simulink model "Grid_FormingVSG_PMSG"  (R2024b)
settings: Solver=ode3  StartTime=0.0  StopTime=44.2  FixedStep=1e-6  RelTol=1e-3  EnableMultiTasking=on
InitFcn:
  | mdlFile = get_param(bdroot,'FileName');
  | mdlDir = fileparts(mdlFile);
  | dtime=4e-6;
  | Ts_step=1e-6;
  | run(fullfile(mdlDir,'GFM_MWT_Nonlinear_Params.m'));
values from neighbouring files (symbols this model uses):
  D_aero = T_aero0 / omega_m0    (= 101321.183642)    [GFM_MWT_Nonlinear_Params.m]    (also in GFM_MWT_Nonlinear_Params_5MW_Liu2024.m = T_aero0/omega_m0)
  D_g = 0.005 * D_aero    (= 506.605918212)    [GFM_MWT_Nonlinear_Params.m]    (also in GFM_MWT_Nonlinear_Params_5MW_Liu2024.m = p5.D_g)
  D_sh = evalin('base','D_sh_override')    [GFM_MWT_Nonlinear_Params.m]    (also in GFM_MWT_Nonlinear_Params_5MW_Liu2024.m = shaft_damping_scale*D_sh)
  D_t = 0.005 * D_aero    (= 506.605918212)    [GFM_MWT_Nonlinear_Params.m]    (also in GFM_MWT_Nonlinear_Params_5MW_Liu2024.m = p5.D_t)
  J_g = 1.83750e5    (= 183750)    [GFM_MWT_Nonlinear_Params.m]    (also in GFM_MWT_Nonlinear_Params_5MW_Liu2024.m = p5.J_g)
  J_t = 8.0 * J_g    (= 1470000)    [GFM_MWT_Nonlinear_Params.m]    (also in GFM_MWT_Nonlinear_Params_5MW_Liu2024.m = p5.J_t)
  K_sh = J_eq * w_sh_init_guess^2    (= 6448141.54205)    [GFM_MWT_Nonlinear_Params.m]    (also in GFM_MWT_Nonlinear_Params_5MW_Liu2024.m = p5.K_sh)
  K_v_aero = 3 * T_aero0 / v_w0    (= 79577.4715459)    [GFM_MWT_Nonlinear_Params.m]    (also in GFM_MWT_Nonlinear_Params_5MW_Liu2024.m = 3*T_aero0/v_w0)
  omega_m0 = 2*pi*30/60    (= 3.14159265359)    [GFM_MWT_Nonlinear_Params.m]    (also in GFM_MWT_Nonlinear_Params_5MW_Liu2024.m = p5.omega_m0)
  T_aero0 = T_e0    (= 318309.886184)    [GFM_MWT_Nonlinear_Params.m]    (also in GFM_MWT_Nonlinear_Params_5MW_Liu2024.m = T_e0)
  theta_tw0 = T_e0 / K_sh    (= 0.0493645935202)    [GFM_MWT_Nonlinear_Params.m]    (also in GFM_MWT_Nonlinear_Params_5MW_Liu2024.m = T_e0/K_sh)
  v_w0 = 12.0    (= 12)    [GFM_MWT_Nonlinear_Params.m]    (also in GFM_MWT_Nonlinear_Params_5MW_Liu2024.m = p5.v_w0)
  wind_step_mps = evalin('base','wind_step_mps_override')    [GFM_MWT_Nonlinear_Params.m]    (also in GFM_MWT_Nonlinear_Params_5MW_Liu2024.m)
  wind_step_time = 1.50    (= 1.5)    [GFM_MWT_Nonlinear_Params.m]    (also in GFM_MWT_Nonlinear_Params_5MW_Liu2024.m = evalin('base','wind_step_time_override'))
undefined symbols (not defined in the file or in its folder): DiscIntNeverNeededParam
libraries: spsSeriesRLCBranchLib x10, spsVoltageMeasurementLib x7, spsCurrentMeasurementLib x6, spsACVoltageSourceLib x3, spsUniversalBridgeLib x2, powerlib_extras x2, spsControlledCurrentSourceLib x2, spsGroundLib x1, simulink x1, spsThreePhaseBreakerLib x1, spspowerguiLib x1
settings Model: Creator=Administrator  LastModifiedBy=Lenovo
settings SolverCC: AlgebraicLoopSolver=TrustRegion
settings DataIOCC: LimitDataPoints=on  LoadInitialState=on  SaveFinalState=on  SaveFormat=Array  SignalLoggingSaveFormat=ModelDataLogs
settings OptimizationCC: ExpressionDepthLimit=2147483647  LifeSpan=inf
settings DebuggingCC: UnderspecifiedInitializationDetection=Classic  MergeDetectMultiDrivingBlocksExec=none  SolverPrmCheckMsg=warning  FcnCallInpInsideContextMsg=warning  UnconnectedInputMsg=warning  UnconnectedOutputMsg=warning  UnconnectedLineMsg=warning  StateNameClashWarn=warning  SFUnexpectedBacktrackingDiag=warning  SFNoUnconditionalDefaultTransitionDiag=warning  SFExecutionAtInitializationDiag=none  ArithmeticOperatorsInVariantConditions=warning
settings HardwareCC: ProdBitPerPointer=32  ProdBitPerSizeT=32  ProdBitPerPtrDiffT=32  ProdLargestAtomicFloat=None  ProdIntDivRoundTo=Undefined  ProdEndianess=Unspecified  ProdWordSize=32  ProdHWDeviceType=32-bit Generic
settings ModelReferenceCC: EnableRefExpFcnMdlSchedulingChecks=on  PropagateSignalLabelsOutOfModel=off
settings SFSimCC: SimUseLocalCustomCode=off  CustomCodeUndefinedFunction=UseInterfaceOnly
settings RTWCC: RTWUseLocalCustomCode=off  GPUComputeCapability=3.5
settings CodeAppCC: StateflowObjectComments=on
settings GRTTargetCC: TargetLangStandard=C89/C90 (ANSI)
settings ConfigComp: CovMetricSettings=dw  CovSaveCumulativeToWorkspaceVar=on  CovSaveSingleToWorkspaceVar=on  CovExternalEMLEnable=off
settings SimscapeCC: SimscapeNormalizeSystem=off

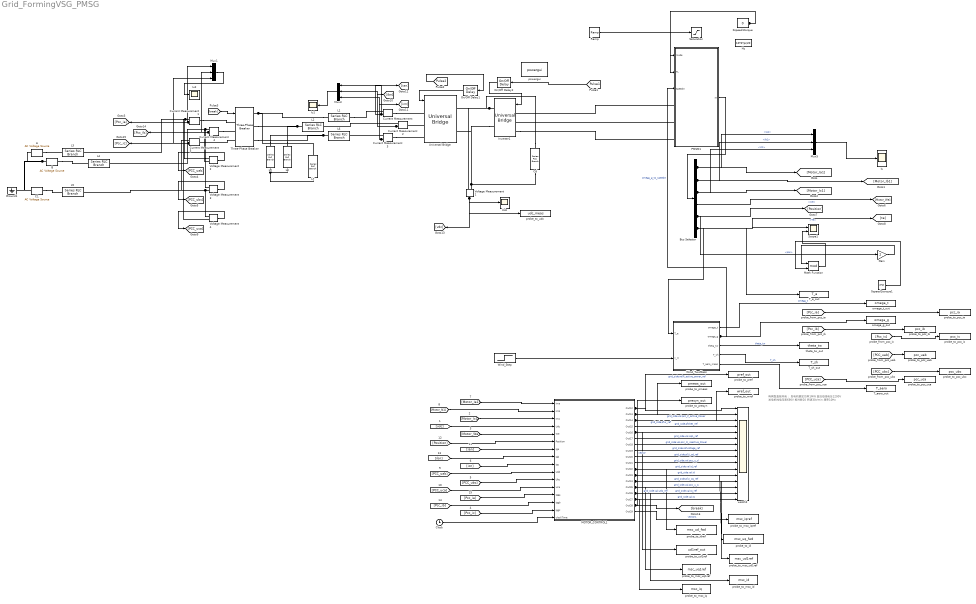
== system Grid_FormingVSG_PMSG ==
  note: 构网型直驱风电：
      | 发电机额定功率1MW
      | 直流母线电压1200V
      | 发电机线电压是690V
      | 极对数20
      | 转速30r/min
      | 频率10Hz
  0speed1torque : Constant  Value=0
  0speed1torque1 : Constant  Value=2*pi
  A : spsACVoltageSourceLib/AC Voltage Source  Amplitude=563  Phase=10  Frequency=50  SampleTime=0  Measurements=None  BusType=swing  Pref=10e3  Qref=0  Qmin=-inf  Qmax=+inf
  B : spsACVoltageSourceLib/AC Voltage Source  Amplitude=563  Phase=-110  Frequency=50  SampleTime=0  Measurements=None  BusType=swing  Pref=10e3  Qref=0  Qmin=-inf  Qmax=+inf
  Bus Selector : BusSelector  OutputSignals=Statormeasurements.ia1,Statormeasurements.ib1,Statormeasurements.ic1,Mechanical.we,Mechanical.pos,Mechanical.Te
  C1 : spsACVoltageSourceLib/AC Voltage Source  Amplitude=563  Phase=130  Frequency=50  SampleTime=0  Measurements=None  BusType=swing  Pref=10e3  Qref=0  Qmin=-inf  Qmax=+inf
  Cd : spsSeriesRLCBranchLib/Series RLC Branch  LConnTagsString=__new0  RConnTagsString=__new0  BranchType=C  Resistance=100  Inductance=1e-3  SetiL0=off  InitialCurrent=0  Capacitance=0.03  Setx0=on  InitialVoltage=1200  Measurements=None
  Clock : Clock
  Current Measurement{,1..5} (6 alike) : spsCurrentMeasurementLib/Current Measurement  PhasorSimulation=off  OutputType=Complex  PSBequivalent=0
  Gain : Gain  Gain=2
  Ground1 : spsGroundLib/Ground  LConnTagsString=a
  Hz : Constant  Value=10*2*pi/20
  Inverter1 : spsUniversalBridgeLib/Universal Bridge  Arms=3  SnubberResistance=1e5  SnubberCapacitance=inf  Device=IGBT / Diodes  Ron=1e-3  Lon=0  ForwardVoltages="[0  0]"  ForwardVoltage=0  GTOparameters=[ 10e-6 , 20e-6 ]  IGBTparameters=[ 1e-6 , 2e-6 ]  Measurements=None  Measurements_2=None  converterType=Rectifier
  Iu : Scope
  Iu1 : Scope
  Iu2 : Scope
  L1 : spsSeriesRLCBranchLib/Series RLC Branch  LConnTagsString=__new0  RConnTagsString=__new0  BranchType=RL  Resistance=0.0002  Inductance=120e-6  SetiL0=off  InitialCurrent=0  Capacitance=2e-3  Setx0=off  InitialVoltage=0  Measurements=None
  L2 : spsSeriesRLCBranchLib/Series RLC Branch  LConnTagsString=__new0  RConnTagsString=__new0  BranchType=RL  Resistance=0.0002  Inductance=120e-6  SetiL0=off  InitialCurrent=0  Capacitance=2e-3  Setx0=off  InitialVoltage=0  Measurements=None
  L3 : spsSeriesRLCBranchLib/Series RLC Branch  LConnTagsString=__new0  RConnTagsString=__new0  BranchType=L  Resistance=0.0083  Inductance=0.48e-3  SetiL0=off  InitialCurrent=0  Capacitance=2e-3  Setx0=off  InitialVoltage=0  Measurements=None
  L4 : spsSeriesRLCBranchLib/Series RLC Branch  LConnTagsString=__new0  RConnTagsString=__new0  BranchType=L  Resistance=0.0083  Inductance=0.48e-3  SetiL0=off  InitialCurrent=0  Capacitance=2e-3  Setx0=off  InitialVoltage=0  Measurements=None
  L5 : spsSeriesRLCBranchLib/Series RLC Branch  LConnTagsString=__new0  RConnTagsString=__new0  BranchType=L  Resistance=0.1  Inductance=0.48e-3  SetiL0=off  InitialCurrent=0  Capacitance=2e-3  Setx0=off  InitialVoltage=0  Measurements=None
  L6 : spsSeriesRLCBranchLib/Series RLC Branch  LConnTagsString=__new0  RConnTagsString=__new0  BranchType=RL  Resistance=0.0002  Inductance=120e-6  SetiL0=off  InitialCurrent=0  Capacitance=2e-3  Setx0=off  InitialVoltage=0  Measurements=None
  L7 : spsSeriesRLCBranchLib/Series RLC Branch  LConnTagsString=__new0  RConnTagsString=__new0  BranchType=C  Resistance=0.0002  Inductance=0.00025  SetiL0=off  InitialCurrent=0  Capacitance=55e-6  Setx0=off  InitialVoltage=0  Measurements=None
  L8 : spsSeriesRLCBranchLib/Series RLC Branch  LConnTagsString=__new0  RConnTagsString=__new0  BranchType=C  Resistance=0.0002  Inductance=0.00025  SetiL0=off  InitialCurrent=0  Capacitance=55e-6  Setx0=off  InitialVoltage=0  Measurements=None
  L9 : spsSeriesRLCBranchLib/Series RLC Branch  LConnTagsString=__new0  RConnTagsString=__new0  BranchType=C  Resistance=0.0002  Inductance=0.00025  SetiL0=off  InitialCurrent=0  Capacitance=55e-6  Setx0=off  InitialVoltage=0  Measurements=None
  MOTOR_CONTROL1 : Subsystem  mask{Pref=1000000, Qref=0, ReferenceACVoltage=563, ReferenceDCVoltage=1000}
      mask prompts: Pref "Active Power"; Qref "Reactive Power"; ReferenceACVoltage "Reference AC Voltage"; ReferenceDCVoltage "Reference DC Voltage"
  Math Function : Math  Operator=mod  SignedPower=on
  Mux1 : Mux  Inputs=3
  Mux3 : Mux  Inputs=3
  Mux5 : Mux  Inputs=3
  On/Off Delay1 : powerlib_extras/Control  Blocks/On//Off Delay  type_delay=On delay  delay=dtime  ic=0
  On/Off Delay2 : powerlib_extras/Control  Blocks/On//Off Delay  type_delay=On delay  delay=dtime  ic=0
  PMSM1 : Subsystem  mask{Rpass=1e2, Cpass=1e-6, Flux=8.64, Rs=0.0122, Lq=0.00105, Ld=0.00105, pairs=20, J=183750, Bw=0.001}
  Ramp : simulink/Sources/Ramp  slope=1000  start=0.2  InitialOutput=0
  Saturation : Saturate  UpperLimit=9.55
  Scope1 : Scope  NumInputPorts=2
  T_aero_out : ToWorkspace  VariableName=T_aero  SaveFormat=Timeseries  SampleTime=-1
      settings: Decimation=mech_log_decimation
  T_e_out : ToWorkspace  VariableName=T_e  SaveFormat=Timeseries  SampleTime=-1
      settings: Decimation=mech_log_decimation
  T_sh_out : ToWorkspace  VariableName=T_sh  SaveFormat=Timeseries  SampleTime=-1
      settings: Decimation=mech_log_decimation
  Three-Phase Breaker : spsThreePhaseBreakerLib/Three-Phase Breaker  InitialState=closed  SwitchA=on  SwitchB=on  SwitchC=on  SwitchTimes=[3 3.15]  External=on  BreakerResistance=0.0001  SnubberResistance=1e6  SnubberCapacitance=inf  Measurements=None
  Udc : Scope
  Universal Bridge : spsUniversalBridgeLib/Universal Bridge  Arms=3  SnubberResistance=1e5  SnubberCapacitance=inf  Device=MOSFET / Diodes  Ron=1e-3  Lon=0  ForwardVoltages="[  0  0  ]"  ForwardVoltage=0  GTOparameters=[ 10e-6 , 20e-6 ]  IGBTparameters=[ 1e-6 , 2e-6 ]  Measurements=None  Measurements_2=None  converterType=Rectifier
  Voltage Measurement{1..4} (4 alike) : spsVoltageMeasurementLib/Voltage Measurement  PhasorSimulation=off  OutputType=Complex  PSBequivalent=0
  Wind_Step : Step  Time=wind_step_time  Before=v_w0  After=v_w0 + wind_step_mps  SampleTime=0
  Wind_TwoMass : Subsystem
  omega_g_out : ToWorkspace  VariableName=omega_g  SaveFormat=Timeseries  SampleTime=-1
      settings: Decimation=mech_log_decimation
  omega_t_out : ToWorkspace  VariableName=omega_t  SaveFormat=Timeseries  SampleTime=-1
      settings: Decimation=mech_log_decimation
  powergui : spspowerguiLib/powergui  SimulationMode=Discrete  SampleTime=Ts_step  frequency=60  Iterations=50  frequencyindice=0  Pbase=100e6  ErrMax=1e-4  UnitsV=kV  UnitsW=MW  buscounter=0  FunctionMessages=off  echomessages=off  EnableUseOfTLC=off  CurrentSourceSwitches=off  DisableSnubberDevices=off  DisableRonSwitches=off  DisableVfSwitches=off  DisplayEquations=off  AutomaticDiscreteSolvers=off  SolverType=Tustin  Interpol=off  ExternalGateDelay=off  methode=off  Ts=0  x0status=blocks  SPID=off  SwTol=0  HookPort=off  NonlinearTolerance=1e-4  nMaxIteration=100  ContinueOnMaxIteration=off  RestoreLinks=warning  ResistiveCurrentMeasurement=off  Frange=[0:2:500]  Ylog=off  Xlog=on  ShowGrid=off  save=off  variable=ZData  structure=Iu1  ZoomFFT=off  StartTime=3.5  cycles=3  DisplayStyle=4  fundamental=50  FreqAxis=off  MaxFrequency=4000  frequencyindicesteady=1  RmsSteady=1  display=off
  probe_to_id : ToWorkspace  VariableName=msc_uq_fwd  SaveFormat=Structure With Time  SampleTime=-1
  probe_to_idref : ToWorkspace  VariableName=msc_ud_fwd  SaveFormat=Structure With Time  SampleTime=-1
  probe_to_msc_id : ToWorkspace  VariableName=msc_id  SaveFormat=Timeseries
  probe_to_msc_iq : ToWorkspace  VariableName=msc_iq  SaveFormat=Timeseries
  probe_to_msc_iqref : ToWorkspace  VariableName=msc_iqref  SaveFormat=Timeseries
  probe_to_msc_ud1ref : ToWorkspace  VariableName=msc_ud1ref  SaveFormat=Timeseries
  probe_to_msc_uq1ref : ToWorkspace  VariableName=msc_uq1ref  SaveFormat=Timeseries
  probe_to_pcc_ia : ToWorkspace  VariableName=pcc_ia  SaveFormat=Timeseries  SampleTime=-1
      settings: Decimation=100
  probe_to_pcc_ib : ToWorkspace  VariableName=pcc_ib  SaveFormat=Timeseries  SampleTime=-1
      settings: Decimation=100
  probe_to_pcc_ic : ToWorkspace  VariableName=pcc_ic  SaveFormat=Timeseries  SampleTime=-1
      settings: Decimation=100
  probe_to_pcc_uab : ToWorkspace  VariableName=pcc_uab  SaveFormat=Timeseries  SampleTime=-1
      settings: Decimation=100
  probe_to_pcc_ubc : ToWorkspace  VariableName=pcc_ubc  SaveFormat=Timeseries  SampleTime=-1
      settings: Decimation=100
  probe_to_pcc_uca : ToWorkspace  VariableName=pcc_uca  SaveFormat=Timeseries  SampleTime=-1
      settings: Decimation=100
  probe_to_pmeas : ToWorkspace  VariableName=pmeas_out  SaveFormat=Timeseries  SampleTime=-1
      settings: Decimation=100
  probe_to_pref : ToWorkspace  VariableName=pref_out  SaveFormat=Timeseries  SampleTime=-1
      settings: Decimation=100
  probe_to_presyn : ToWorkspace  VariableName=presyn_out  SaveFormat=Timeseries  SampleTime=-1
      settings: Decimation=100
  probe_to_ud1ref : ToWorkspace  VariableName=ud1ref_out  SaveFormat=Structure With Time  SampleTime=-1
  probe_to_udc : ToWorkspace  VariableName=udc_meas  SaveFormat=Timeseries  SampleTime=-1
      settings: Decimation=100
  probe_to_wref : ToWorkspace  VariableName=wref_out  SaveFormat=Timeseries  SampleTime=-1
      settings: Decimation=100
  theta_tw_out : ToWorkspace  VariableName=theta_tw  SaveFormat=Timeseries  SampleTime=-1
      settings: Decimation=mech_log_decimation
  watch2 : Scope  NumInputPorts=16
  wires:
  MOTOR_CONTROL1/18(Out29) -> probe_to_msc_iqref/1  "vector1"
  Wind_TwoMass/5(T_aero_meas) -> T_aero_out/1
  [PCC_uca] -> probe_to_pcc_uca/1
  [PCC_ubc] -> probe_to_pcc_ubc/1
  [PCC_uab] -> probe_to_pcc_uab/1
  [Pcc_ic] -> probe_to_pcc_ic/1
  [Pcc_ib] -> probe_to_pcc_ib/1
  [Pcc_ia] -> probe_to_pcc_ia/1
  Wind_TwoMass/4(T_sh) -> T_sh_out/1  "T_sh"
  Wind_TwoMass/3(theta_tw) -> theta_tw_out/1  "theta_tw"
  Wind_TwoMass/1(omega_t) -> omega_t_out/1  "omega_t"
  Wind_TwoMass/2(omega_g) -> PMSM1/3(Speedin), omega_g_out/1  "omega_g_to_speedin"
  Wind_Step/1 -> Wind_TwoMass/2(v_w)
  Current Measurement3/1 -> Mux3/3, [icn]
  Current Measurement2/1 -> [ibn], Mux3/2
  Current Measurement/1 -> [ian], Mux3/1
  Current Measurement5/1 -> [Pcc_ic], Mux1/3
  Current Measurement4/1 -> [Pcc_ib], Mux1/2
  Current Measurement1/1 -> [Pcc_ia], Mux1/1
  Mux1/1 -> Iu2/1
  [break] -> Three-Phase Breaker/1
  MOTOR_CONTROL1/17(Out28) -> probe_to_presyn/1, [break]  "vector"
  Clock/1 -> MOTOR_CONTROL1/16(clockTime)
  [Pcc_ic] -> MOTOR_CONTROL1/15(Iggc)
  [Pcc_ib] -> MOTOR_CONTROL1/14(Iggb)
  [Pcc_ia] -> MOTOR_CONTROL1/13(Igga)
  Voltage Measurement3/1 -> [PCC_ubc]
  Voltage Measurement4/1 -> [PCC_uca]
  Voltage Measurement2/1 -> [PCC_uab]
  [ian] -> MOTOR_CONTROL1/7(Iga)
  [PCC_ubc] -> MOTOR_CONTROL1/11(Ubc)
  [PCC_uca] -> MOTOR_CONTROL1/12(Uca)
  [ibn] -> MOTOR_CONTROL1/8(Igb)
  [PCC_uab] -> MOTOR_CONTROL1/10(Uab)
  [icn] -> MOTOR_CONTROL1/9(Igc)
  On/Off Delay1/1 -> Universal Bridge/1
  [Pulse2] -> On/Off Delay1/1
  Mux3/1 -> Iu1/1
  Voltage Measurement1/1 -> Udc/1, [vdc], probe_to_udc/1
  [Motor_Ia1] -> MOTOR_CONTROL1/1(Ima)
  MOTOR_CONTROL1/8(Out19) -> watch2/8  "grid_side.ref.voltage_ref"
  MOTOR_CONTROL1/6(Out17) -> watch2/6  "grid_side.val.Uq1_ref"
  [vdc] -> MOTOR_CONTROL1/4(Udc)
  [Motor_Ic1] -> MOTOR_CONTROL1/3(Imc)
  [Position] -> MOTOR_CONTROL1/6(Position)
  MOTOR_CONTROL1/1(Out12) -> probe_to_pref/1, watch2/1  "grid_side.ref.P_active_power_ref"
  MOTOR_CONTROL1/2(Out13) -> probe_to_pmeas/1, watch2/2  "grid_side.val.pcc_P_active_Power"
  MOTOR_CONTROL1/11(Out22) -> probe_to_idref/1, watch2/11  "grid_side.val.Id_ref"
  MOTOR_CONTROL1/4(Out15) -> watch2/4  "grid_side.pf.thet_ref"
  MOTOR_CONTROL1/16(Out27) -> probe_to_msc_iq/1, watch2/16  "grid_side.val.Iq"
  MOTOR_CONTROL1/3(Out14) -> probe_to_wref/1, watch2/3  "grid_side.pf.w_ref"
  MOTOR_CONTROL1/9(Out20) -> watch2/9  "grid_side.pf.U_od_ref"
  MOTOR_CONTROL1/10(Out21) -> watch2/10  "grid_side.val.pcc_u_d"
  MOTOR_CONTROL1/15(Out26) -> probe_to_msc_id/1, watch2/15  "grid_side.val.Iq_ref"
  [Motor_We] -> MOTOR_CONTROL1/5(We)
  MOTOR_CONTROL1/14(Out25) -> probe_to_msc_uq1ref/1, watch2/14  "grid_side.val.pcc_u_q"
  MOTOR_CONTROL1/5(Out16) -> probe_to_ud1ref/1, watch2/5  "grid_side.val.Ud1_ref"
  MOTOR_CONTROL1/7(Out18) -> watch2/7  "grid_side.val.pcc_Q_reactive_Power"
  MOTOR_CONTROL1/13(Out24) -> watch2/13, probe_to_msc_ud1ref/1  "grid_side.pf.U_oq_ref"
  [Motor_Ib1] -> MOTOR_CONTROL1/2(Imb)
  MOTOR_CONTROL1/12(Out23) -> probe_to_id/1, watch2/12  "grid_side.val.Id"
  0speed1torque1/1 -> Math Function/2
  0speed1torque/1 -> PMSM1/1(mode), PMSM1/2(TL)
  Mux5/1 -> Iu/1
  Bus Selector/4 -> [Motor_We]  "<we>"
  Gain/1 -> Math Function/1
  Bus Selector/1 -> [Motor_Ia1], Mux5/1  "<ia1>"
  PMSM1/1(M) -> Bus Selector/1
  Bus Selector/2 -> [Motor_Ib1], Mux5/2  "<ib1>"
  Bus Selector/6 -> [te], Scope1/1, Wind_TwoMass/1(T_e), T_e_out/1  "<Te>"
  Ramp/1 -> Saturation/1
  Math Function/1 -> Scope1/2
  Bus Selector/3 -> [Motor_Ic1], Mux5/3  "<ic1>"
  Bus Selector/5 -> [Position], Gain/1  "<pos>"
  On/Off Delay2/1 -> Inverter1/1
  [Pulse1] -> On/Off Delay2/1
  connections:
  L1/RConn1 -- Current Measurement/RConn1
  Current Measurement2/RConn1 -- L2/RConn1
  Current Measurement3/RConn1 -- L6/RConn1
  Current Measurement3/LConn1 -- Universal Bridge/LConn3
  Universal Bridge/LConn2 -- Current Measurement2/LConn1
  Current Measurement/LConn1 -- Universal Bridge/LConn1
  Three-Phase Breaker/LConn3 -- Current Measurement5/LConn1
  Current Measurement4/LConn1 -- Three-Phase Breaker/LConn2
  Current Measurement1/LConn1 -- Three-Phase Breaker/LConn1
  Cd/LConn1 -- Inverter1/RConn1 -- Universal Bridge/RConn1 -- Voltage Measurement1/LConn1
  L8/LConn1 -- Three-Phase Breaker/RConn2 -- L2/LConn1
  L1/LConn1 -- L7/LConn1 -- Three-Phase Breaker/RConn1
  L9/LConn1 -- Three-Phase Breaker/RConn3 -- L6/LConn1
  L7/RConn1 -- L8/RConn1 -- L9/RConn1
  Voltage Measurement4/LConn1 -- Voltage Measurement3/LConn2 -- Current Measurement5/RConn1 -- L5/RConn1
  Voltage Measurement3/LConn1 -- Voltage Measurement2/LConn2 -- Current Measurement4/RConn1 -- L4/RConn1
  A/RConn1 -- L3/LConn1
  Voltage Measurement2/LConn1 -- Voltage Measurement4/LConn2 -- Current Measurement1/RConn1 -- L3/RConn1
  C1/RConn1 -- L5/LConn1
  B/RConn1 -- L4/LConn1
  Inverter1/RConn2 -- Cd/RConn1 -- Voltage Measurement1/LConn2 -- Universal Bridge/RConn2
  B/LConn1 -- C1/LConn1 -- Ground1/LConn1 -- A/LConn1
  Inverter1/LConn3 -- PMSM1/LConn3
  PMSM1/LConn2 -- Inverter1/LConn2
  PMSM1/LConn1 -- Inverter1/LConn1

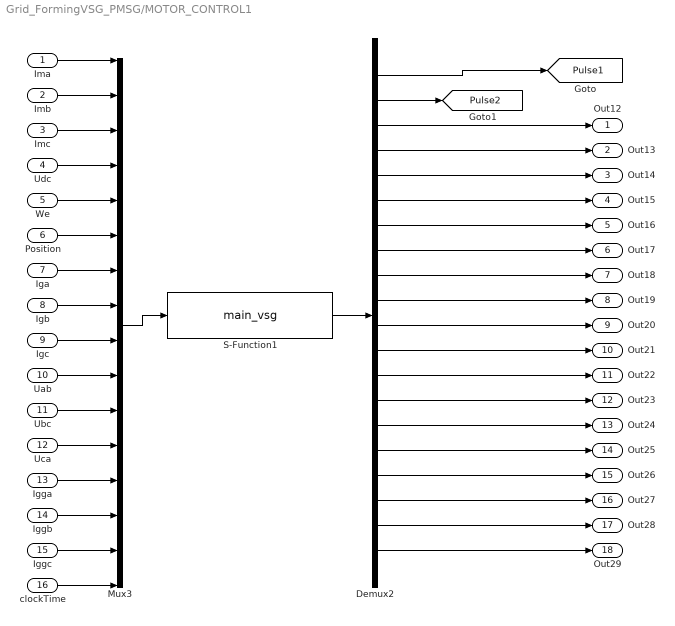
== system Grid_FormingVSG_PMSG/MOTOR_CONTROL1 ==
  Ima : Inport
  Imb : Inport  Port=2
  Imc : Inport  Port=3
  Udc : Inport  Port=4
  We : Inport  Port=5
  Position : Inport  Port=6
  Iga : Inport  Port=7
  Igb : Inport  Port=8
  Igc : Inport  Port=9
  Uab : Inport  Port=10
  Ubc : Inport  Port=11
  Uca : Inport  Port=12
  Igga : Inport  Port=13
  Iggb : Inport  Port=14
  Iggc : Inport  Port=15
  clockTime : Inport  Port=16
  Demux2 : Demux  Outputs=[6 6 1 1 1 1 1 1 1 1 1 1 1 1 1 1 1 1 1 1]
      settings: DisplayOption=none
  Mux3 : Mux  Inputs=16
  S-Function1 : S-Function  FunctionName=main_vsg  Parameters=1000000, 0, 563, 1000  SFunctionDeploymentMode=off  EnableBusSupport=off
  Out12 : Outport  VectorParamsAs1DForOutWhenUnconnected=off
  Out13 : Outport  Port=2  VectorParamsAs1DForOutWhenUnconnected=off
  Out14 : Outport  Port=3  VectorParamsAs1DForOutWhenUnconnected=off
  Out15 : Outport  Port=4  VectorParamsAs1DForOutWhenUnconnected=off
  Out16 : Outport  Port=5  VectorParamsAs1DForOutWhenUnconnected=off
  Out17 : Outport  Port=6  VectorParamsAs1DForOutWhenUnconnected=off
  Out18 : Outport  Port=7  VectorParamsAs1DForOutWhenUnconnected=off
  Out19 : Outport  Port=8  VectorParamsAs1DForOutWhenUnconnected=off
  Out20 : Outport  Port=9  VectorParamsAs1DForOutWhenUnconnected=off
  Out21 : Outport  Port=10  VectorParamsAs1DForOutWhenUnconnected=off
  Out22 : Outport  Port=11  VectorParamsAs1DForOutWhenUnconnected=off
  Out23 : Outport  Port=12  VectorParamsAs1DForOutWhenUnconnected=off
  Out24 : Outport  Port=13  VectorParamsAs1DForOutWhenUnconnected=off
  Out25 : Outport  Port=14  VectorParamsAs1DForOutWhenUnconnected=off
  Out26 : Outport  Port=15  VectorParamsAs1DForOutWhenUnconnected=off
  Out27 : Outport  Port=16  VectorParamsAs1DForOutWhenUnconnected=off
  Out28 : Outport  Port=17  VectorParamsAs1DForOutWhenUnconnected=off
  Out29 : Outport  Port=18  VectorParamsAs1DForOutWhenUnconnected=off
  tag scope: Pulse1=global, Pulse2=global
  wires:
  S-Function1/1 -> Demux2/1
  Demux2/1 -> [Pulse1]
  Demux2/3 -> Out12/1
  Demux2/4 -> Out13/1
  Demux2/5 -> Out14/1
  Demux2/6 -> Out15/1
  Demux2/7 -> Out16/1
  Demux2/8 -> Out17/1
  Demux2/9 -> Out18/1
  Demux2/10 -> Out19/1
  Demux2/11 -> Out20/1
  Demux2/12 -> Out21/1
  Demux2/13 -> Out22/1
  Demux2/14 -> Out23/1
  Demux2/15 -> Out24/1
  Demux2/16 -> Out25/1
  Demux2/17 -> Out26/1
  Demux2/18 -> Out27/1
  Demux2/19 -> Out28/1
  Demux2/20 -> Out29/1
  Imb/1 -> Mux3/2
  Ima/1 -> Mux3/1
  Imc/1 -> Mux3/3
  We/1 -> Mux3/5
  Mux3/1 -> S-Function1/1
  Demux2/2 -> [Pulse2]
  Udc/1 -> Mux3/4
  Position/1 -> Mux3/6
  Uab/1 -> Mux3/10
  Ubc/1 -> Mux3/11
  Iga/1 -> Mux3/7
  Igb/1 -> Mux3/8
  Uca/1 -> Mux3/12
  Igc/1 -> Mux3/9
  Iggc/1 -> Mux3/15
  Iggb/1 -> Mux3/14
  Igga/1 -> Mux3/13
  clockTime/1 -> Mux3/16

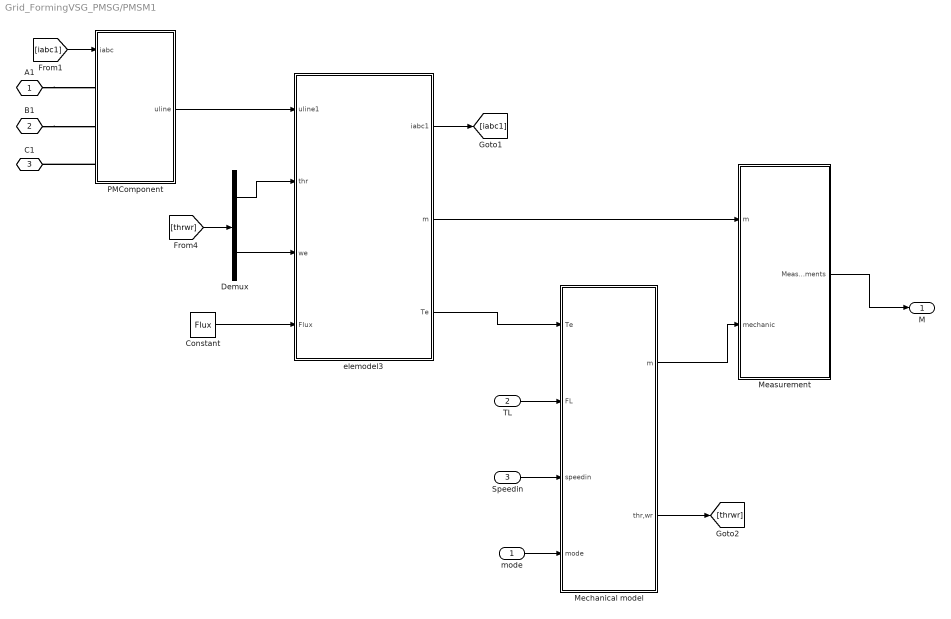
== system Grid_FormingVSG_PMSG/PMSM1 ==
  mode : Inport
  TL : Inport  Port=2
  Speedin : Inport  Port=3
  Constant : Constant  Value=Flux
  Demux : Demux  Outputs=2
  Measurement : Subsystem
  Mechanical model : Subsystem
  PMComponent : Subsystem
  elemodel3 : Subsystem
  A1 : PMIOPort  Side=Left
  B1 : PMIOPort  Port=2  Side=Left
  C1 : PMIOPort  Port=3  Side=Left
  M : Outport  VectorParamsAs1DForOutWhenUnconnected=off
  wires:
  PMComponent/1(uline) -> elemodel3/1(uline1)
  Constant/1 -> elemodel3/4(Flux)
  Mechanical model/2(thr,wr) -> [thrwr]
  [thrwr] -> Demux/1
  Measurement/1(Measurements) -> M/1
  Mechanical model/1(m) -> Measurement/2(mechanic)
  TL/1 -> Mechanical model/2(FL)
  Speedin/1 -> Mechanical model/3(speedin)
  mode/1 -> Mechanical model/4(mode)
  elemodel3/3(Te) -> Mechanical model/1(Te)
  elemodel3/2(m) -> Measurement/1(m)
  Demux/1 -> elemodel3/2(thr)
  Demux/2 -> elemodel3/3(we)
  elemodel3/1(iabc1) -> [iabc1]
  [iabc1] -> PMComponent/1(iabc)
  connections:
  A1/RConn1 -- PMComponent/LConn1
  B1/RConn1 -- PMComponent/LConn2
  PMComponent/LConn3 -- C1/RConn1

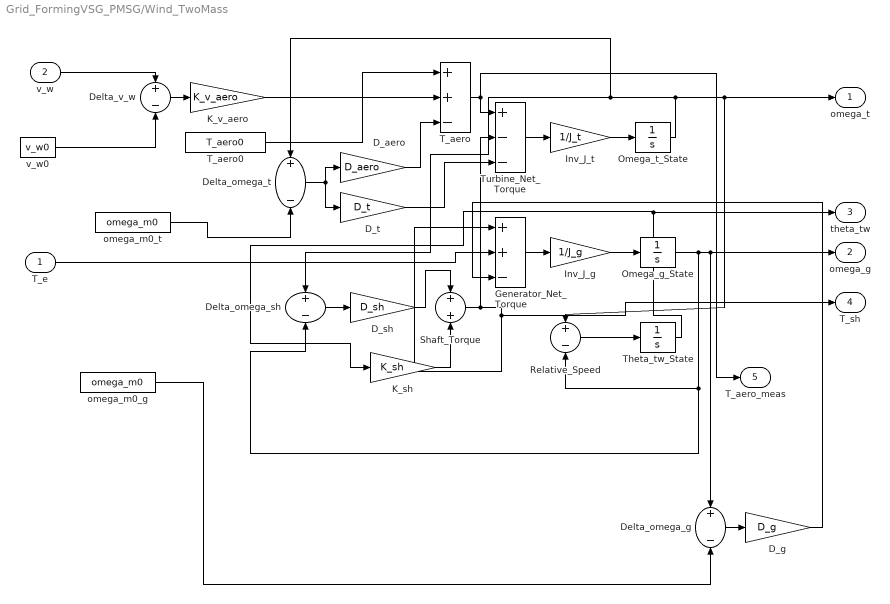
== system Grid_FormingVSG_PMSG/Wind_TwoMass ==
  T_e : Inport
  v_w : Inport  Port=2
  D_aero : Gain  Gain=D_aero
  D_g : Gain  Gain=D_g
  D_sh : Gain  Gain=D_sh
  D_t : Gain  Gain=D_t
  Delta_omega_g : Sum  Inputs=+-
  Delta_omega_sh : Sum  Inputs=+-
  Delta_omega_t : Sum  Inputs=+-
  Delta_v_w : Sum  Inputs=+-
  Generator_Net_Torque : Sum  Inputs=++-
  Inv_J_g : Gain  Gain=1/J_g
  Inv_J_t : Gain  Gain=1/J_t
  K_sh : Gain  Gain=K_sh
  K_v_aero : Gain  Gain=K_v_aero
  Omega_g_State : Integrator  InitialCondition=omega_m0
  Omega_t_State : Integrator  InitialCondition=omega_m0
  Relative_Speed : Sum  Inputs=+-
  Shaft_Torque : Sum
  T_aero : Sum  Inputs=++-
  T_aero0 : Constant  Value=T_aero0
  Theta_tw_State : Integrator  InitialCondition=theta_tw0
  Turbine_Net_Torque : Sum  Inputs=+--
  omega_m0_g : Constant  Value=omega_m0
  omega_m0_t : Constant  Value=omega_m0
  v_w0 : Constant  Value=v_w0
  omega_t : Outport
  omega_g : Outport  Port=2
  theta_tw : Outport  Port=3
  T_sh : Outport  Port=4
  T_aero_meas : Outport  Port=5
  wires:
  v_w/1 -> Delta_v_w/1
  v_w0/1 -> Delta_v_w/2
  Delta_v_w/1 -> K_v_aero/1
  K_v_aero/1 -> T_aero/2
  T_aero0/1 -> T_aero/1
  Omega_t_State/1 -> Relative_Speed/1, omega_t/1, Delta_omega_t/1, Delta_omega_sh/1
  omega_m0_t/1 -> Delta_omega_t/2
  Delta_omega_t/1 -> D_aero/1, D_t/1
  D_aero/1 -> T_aero/3
  Omega_g_State/1 -> omega_g/1, Delta_omega_g/1, Delta_omega_sh/2, Relative_Speed/2
  Delta_omega_sh/1 -> D_sh/1
  Theta_tw_State/1 -> K_sh/1, theta_tw/1
  D_sh/1 -> Shaft_Torque/1
  K_sh/1 -> Shaft_Torque/2
  T_aero/1 -> Turbine_Net_Torque/1, T_aero_meas/1
  Shaft_Torque/1 -> Generator_Net_Torque/1, T_sh/1, Turbine_Net_Torque/2
  D_t/1 -> Turbine_Net_Torque/3
  Turbine_Net_Torque/1 -> Inv_J_t/1
  Inv_J_t/1 -> Omega_t_State/1
  omega_m0_g/1 -> Delta_omega_g/2
  Delta_omega_g/1 -> D_g/1
  T_e/1 -> Generator_Net_Torque/2
  D_g/1 -> Generator_Net_Torque/3
  Generator_Net_Torque/1 -> Inv_J_g/1
  Inv_J_g/1 -> Omega_g_State/1
  Relative_Speed/1 -> Theta_tw_State/1

== system Grid_FormingVSG_PMSG/PMSM1/Measurement ==
  m : Inport
  mechanic : Inport  Port=2
  Bus Creator : BusCreator  Inputs=8
  Bus Creator3 : BusCreator  Inputs=3
  Bus Creator5 : BusCreator  Inputs=2
  Demux : Demux  Outputs=[1,1,1,1,1,1,1,1]
  Demux1 : Demux  Outputs=[1,1,1]
  Measurements : Outport  VectorParamsAs1DForOutWhenUnconnected=off
  wires:
  m/1 -> Demux/1
  Bus Creator5/1 -> Measurements/1
  Demux/1 -> Bus Creator/1  "ia1"
  Demux/2 -> Bus Creator/2  "ib1"
  Demux/8 -> Bus Creator/8  "vc1"
  Demux/3 -> Bus Creator/3  "ic1"
  Bus Creator/1 -> Bus Creator5/1  "Statormeasurements"
  Bus Creator3/1 -> Bus Creator5/2  "Mechanical"
  ? -> ?  "fluxd"
  ? -> ?  "fluxq"
  mechanic/1 -> Demux1/1
  Demux1/1 -> Bus Creator3/1  "we"
  Demux1/2 -> Bus Creator3/2  "pos"
  Demux1/3 -> Bus Creator3/3  "Te"
  Demux/4 -> Bus Creator/4  "fluxd"
  Demux/5 -> Bus Creator/5  "fluxq"
  Demux/6 -> Bus Creator/6  "va1"
  Demux/7 -> Bus Creator/7  "vb1"

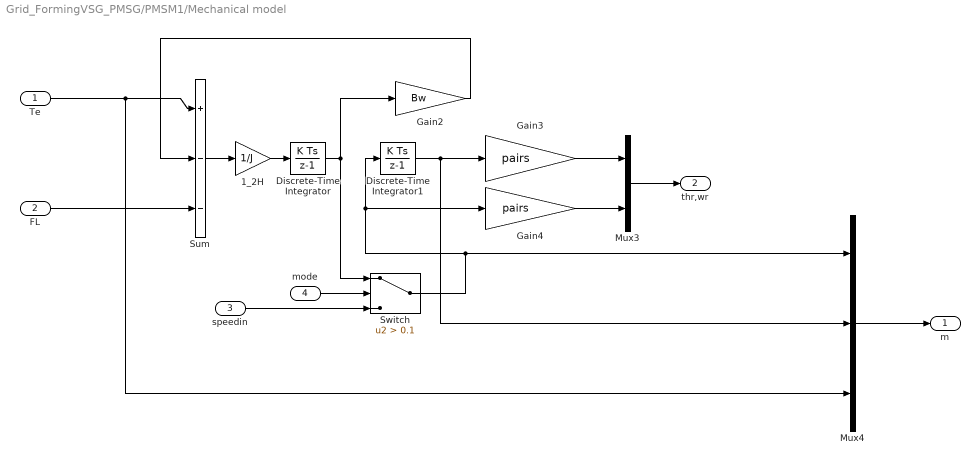
== system Grid_FormingVSG_PMSG/PMSM1/Mechanical model ==
  Te : Inport
  FL : Inport  Port=2
  speedin : Inport  Port=3
  mode : Inport  Port=4
  1_2H : Gain  Gain=1/J  SaturateOnIntegerOverflow=on  OutDataTypeStr=Inherit: Same as input  ParamDataTypeStr=Inherit: Same as input
  Discrete-Time Integrator : DiscreteIntegrator  SampleTime=Ts_step  UpperSaturationLimit=1000000  LowerSaturationLimit=-1000000  ICPrevOutput=DiscIntNeverNeededParam  ICPrevScaledInput=DiscIntNeverNeededParam
  Discrete-Time Integrator1 : DiscreteIntegrator  SampleTime=Ts_step  ICPrevOutput=DiscIntNeverNeededParam  ICPrevScaledInput=DiscIntNeverNeededParam
  Gain2 : Gain  Gain=Bw
  Gain3 : Gain  Gain=pairs
  Gain4 : Gain  Gain=pairs
  Mux3 : Mux  Inputs=2
  Mux4 : Mux  Inputs=3
  Sum : Sum  Inputs=+--  InputSameDT=on  SaturateOnIntegerOverflow=on  OutDataTypeStr=Inherit: Same as first input
  Switch : Switch  Criteria=u2 > Threshold  Threshold=0.1  SaturateOnIntegerOverflow=off  InputSameDT=off
  m : Outport  VectorParamsAs1DForOutWhenUnconnected=off
  thr,wr : Outport  Port=2  VectorParamsAs1DForOutWhenUnconnected=off
  wires:
  Mux4/1 -> m/1
  Mux3/1 -> thr,wr/1
  Te/1 -> Sum/1, Mux4/3
  Sum/1 -> 1_2H/1
  Discrete-Time Integrator/1 -> Gain2/1, Switch/1
  Discrete-Time Integrator1/1 -> Gain3/1, Mux4/2
  1_2H/1 -> Discrete-Time Integrator/1
  Gain3/1 -> Mux3/1
  Gain4/1 -> Mux3/2
  mode/1 -> Switch/2
  speedin/1 -> Switch/3
  Switch/1 -> Discrete-Time Integrator1/1, Gain4/1, Mux4/1
  FL/1 -> Sum/3
  Gain2/1 -> Sum/2

== system Grid_FormingVSG_PMSG/PMSM1/PMComponent ==
  iabc : Inport
  CURRENT INJECTION SYSTEM : Subsystem
  MEASUREMENT SYSTEM : Subsystem
  A1 : PMIOPort  Side=Left
  B1 : PMIOPort  Port=2  Side=Left
  C1 : PMIOPort  Port=3  Side=Left
  uline : Outport  VectorParamsAs1DForOutWhenUnconnected=off
  wires:
  iabc/1 -> CURRENT INJECTION SYSTEM/1(currents)
  MEASUREMENT SYSTEM/1(u_line) -> uline/1
  connections:
  B1/RConn1 -- MEASUREMENT SYSTEM/LConn2 -- CURRENT INJECTION SYSTEM/RConn2
  A1/RConn1 -- CURRENT INJECTION SYSTEM/RConn1 -- MEASUREMENT SYSTEM/LConn1
  MEASUREMENT SYSTEM/LConn3 -- C1/RConn1 -- CURRENT INJECTION SYSTEM/RConn3

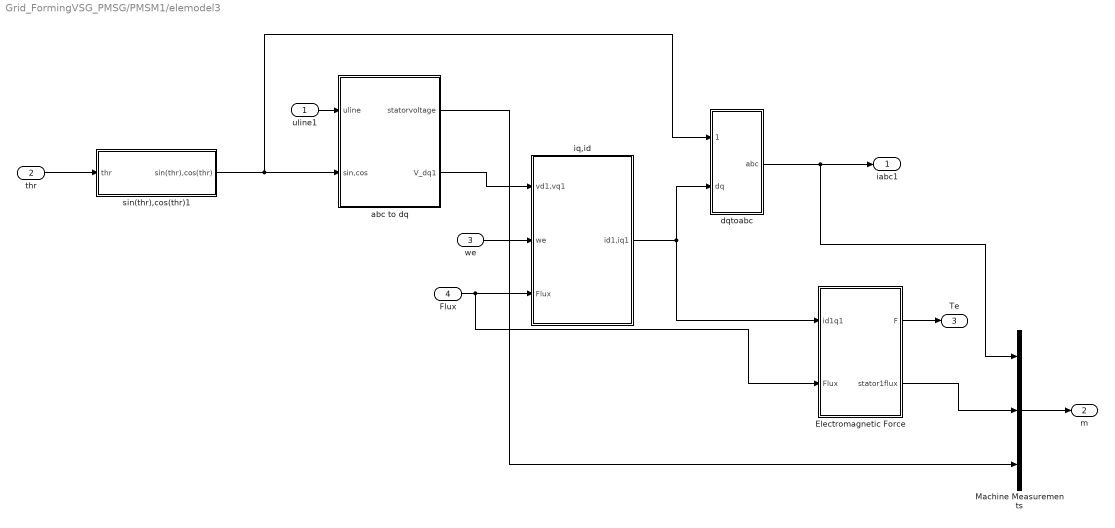
== system Grid_FormingVSG_PMSG/PMSM1/elemodel3 ==
  uline1 : Inport
  thr : Inport  Port=2
  we : Inport  Port=3
  Flux : Inport  Port=4
  Electromagnetic Force : Subsystem  AncestorBlock=|
      | spsSynchronousMachineModel/Continuous/Synchronous Machine
      | Continuous Model/Electromagnetic
      | Torque
  Machine Measurements : Mux  Inputs=[3,2,3]
  abc to dq : Subsystem  AncestorBlock="spsAsynchronousMachineModel/Continuous/abc to dq  transformation"
      mask Display: disp('abc2qd')
  dqtoabc : Subsystem
  iq,id : Subsystem  AncestorBlock=spsPMSynchronousMachineModel/Continuous/iq,id
  sin(thr),cos(thr)1 : Subsystem  TreatAsAtomicUnit=on
  iabc1 : Outport  VectorParamsAs1DForOutWhenUnconnected=off
  m : Outport  Port=2  VectorParamsAs1DForOutWhenUnconnected=off
  Te : Outport  Port=3  VectorParamsAs1DForOutWhenUnconnected=off
  wires:
  sin(thr),cos(thr)1/1(sin(thr),cos(thr)) -> abc to dq/2(sin,cos), dqtoabc/1(sincos)
  abc to dq/2(V_dq1) -> iq,id/1(vd1,vq1)
  Electromagnetic Force/1(F) -> Te/1
  uline1/1 -> abc to dq/1(uline)
  thr/1 -> sin(thr),cos(thr)1/1(thr)
  we/1 -> iq,id/2(we)
  Flux/1 -> iq,id/3(Flux), Electromagnetic Force/2(Flux)
  iq,id/1(id1,iq1) -> dqtoabc/2(dq), Electromagnetic Force/1(id1q1)
  dqtoabc/1(abc) -> iabc1/1, Machine Measurements/1
  Machine Measurements/1 -> m/1
  Electromagnetic Force/2(stator1flux) -> Machine Measurements/2
  abc to dq/1(statorvoltage) -> Machine Measurements/3

== system Grid_FormingVSG_PMSG/PMSM1/PMComponent/CURRENT INJECTION SYSTEM ==
  currents : Inport
  Controlled Current Source : spsControlledCurrentSourceLib/Controlled Current Source  Initialize=on  Source_Type=AC  Amplitude=0  Phase=0  Frequency=0  Measurements=None
  Controlled Current Source1 : spsControlledCurrentSourceLib/Controlled Current Source  Initialize=on  Source_Type=AC  Amplitude=0  Phase=0  Frequency=0  Measurements=None
  Demux : Demux  Outputs=2
  Selector : Selector  InputPortWidth=3  IndexOptions=Index vector (dialog)  Indices=1:2  OutputSizes=1
  A1 : PMIOPort  Side=Right
  B1 : PMIOPort  Port=2  Side=Right
  C1 : PMIOPort  Port=3  Side=Right
  wires:
  Demux/1 -> Controlled Current Source/1
  Demux/2 -> Controlled Current Source1/1
  currents/1 -> Selector/1
  Selector/1 -> Demux/1
  connections:
  Controlled Current Source/LConn1 -- A1/RConn1
  Controlled Current Source1/LConn1 -- B1/RConn1
  Controlled Current Source/RConn1 -- Controlled Current Source1/RConn1 -- C1/RConn1

== system Grid_FormingVSG_PMSG/PMSM1/PMComponent/MEASUREMENT SYSTEM ==
  Mux : Mux  Inputs=3
  V_AB : spsVoltageMeasurementLib/Voltage Measurement  PhasorSimulation=off  OutputType=Complex  PSBequivalent=0
  V_BC : spsVoltageMeasurementLib/Voltage Measurement  PhasorSimulation=off  OutputType=Complex  PSBequivalent=0
  V_CA : spsVoltageMeasurementLib/Voltage Measurement  PhasorSimulation=off  OutputType=Complex  PSBequivalent=0
  A1 : PMIOPort  Side=Left
  B1 : PMIOPort  Port=2  Side=Left
  C1 : PMIOPort  Port=3  Side=Left
  u_line : Outport  VectorParamsAs1DForOutWhenUnconnected=off
  wires:
  Mux/1 -> u_line/1
  V_BC/1 -> Mux/2
  V_AB/1 -> Mux/1
  V_CA/1 -> Mux/3
  connections:
  V_AB/LConn1 -- A1/RConn1 -- V_CA/LConn2
  V_BC/LConn2 -- C1/RConn1 -- V_CA/LConn1
  V_BC/LConn1 -- V_AB/LConn2 -- B1/RConn1

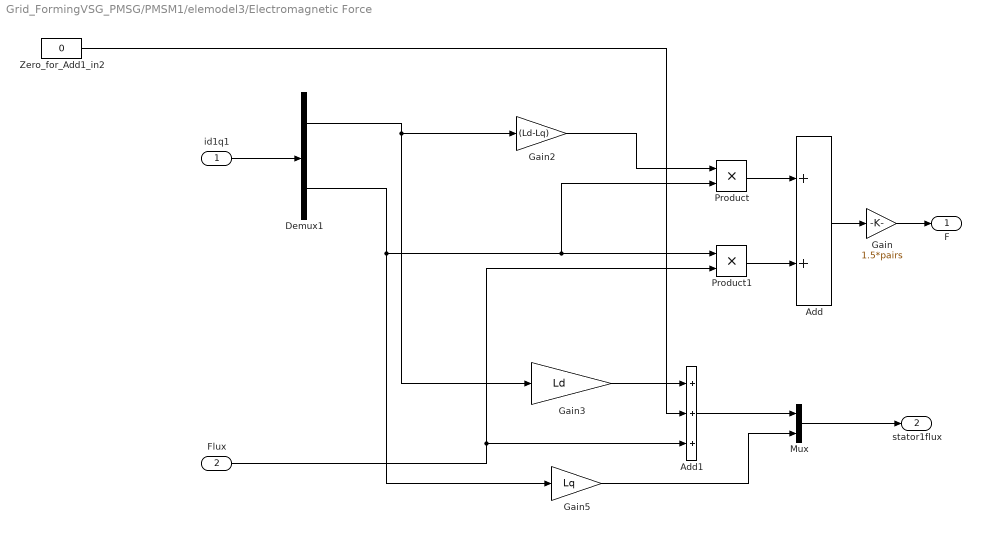
== system Grid_FormingVSG_PMSG/PMSM1/elemodel3/Electromagnetic Force ==
  id1q1 : Inport
  Flux : Inport  Port=2
  Add : Sum
  Add1 : Sum  Inputs=+++
  Demux1 : Demux  Outputs=2
  Gain : Gain  Gain=1.5*pairs
  Gain2 : Gain  Gain=(Ld-Lq)
  Gain3 : Gain  Gain=Ld
  Gain5 : Gain  Gain=Lq
  Mux : Mux  Inputs=2
  Product : Product  RndMeth=Zero
  Product1 : Product  RndMeth=Zero
  Zero_for_Add1_in2 : Constant  Value=0
  F : Outport  VectorParamsAs1DForOutWhenUnconnected=off
  stator1flux : Outport  Port=2  VectorParamsAs1DForOutWhenUnconnected=off
  wires:
  id1q1/1 -> Demux1/1
  Add/1 -> Gain/1
  Product/1 -> Add/1
  Product1/1 -> Add/2
  Gain/1 -> F/1
  Gain3/1 -> Add1/1
  Add1/1 -> Mux/1
  Mux/1 -> stator1flux/1
  Flux/1 -> Product1/2, Add1/3
  Demux1/2 -> Product1/1, Product/2, Gain5/1
  Demux1/1 -> Gain2/1, Gain3/1
  Gain2/1 -> Product/1
  Gain5/1 -> Mux/2
  Zero_for_Add1_in2/1 -> Add1/2

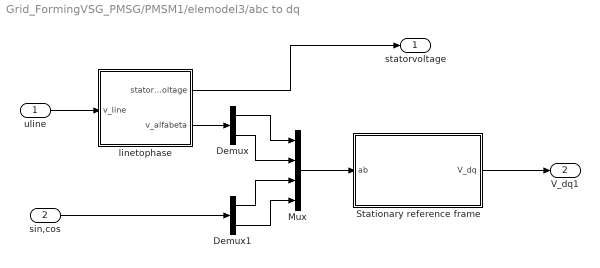
== system Grid_FormingVSG_PMSG/PMSM1/elemodel3/abc to dq ==
  uline : Inport
  sin,cos : Inport  Port=2
  Demux : Demux  Outputs=2
  Demux1 : Demux  Outputs=2
  Mux : Mux
  Stationary reference frame : Subsystem  AncestorBlock="spsAsynchronousMachineModel/Continuous/abc to dq  transformation/Stationary reference frame"  TreatAsAtomicUnit=on
      mask Display: disp('Stationary\nreference\nframe')
  linetophase : Subsystem
  statorvoltage : Outport  VectorParamsAs1DForOutWhenUnconnected=off
  V_dq1 : Outport  Port=2  VectorParamsAs1DForOutWhenUnconnected=off
  wires:
  uline/1 -> linetophase/1(v_line)
  Stationary reference frame/1(V_dq) -> V_dq1/1
  linetophase/2(v_alfabeta) -> Demux/1
  sin,cos/1 -> Demux1/1
  Demux/1 -> Mux/1
  Demux/2 -> Mux/2
  Demux1/1 -> Mux/3
  Demux1/2 -> Mux/4
  Mux/1 -> Stationary reference frame/1(ab)
  linetophase/1(stator_voltage) -> statorvoltage/1

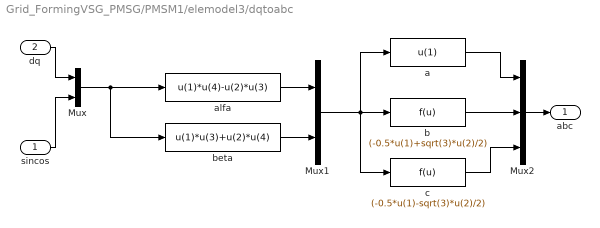
== system Grid_FormingVSG_PMSG/PMSM1/elemodel3/dqtoabc ==
  sincos : Inport
  dq : Inport  Port=2
  Mux : Mux  Inputs=2
  Mux1 : Mux  Inputs=2
  Mux2 : Mux  Inputs=3
  a : Fcn  Expr=u(1)
  alfa : Fcn  Expr=u(1)*u(4)-u(2)*u(3)
  b : Fcn  Expr=(-0.5*u(1)+sqrt(3)*u(2)/2)
  beta : Fcn  Expr=u(1)*u(3)+u(2)*u(4)
  c : Fcn  Expr=(-0.5*u(1)-sqrt(3)*u(2)/2)
  abc : Outport  VectorParamsAs1DForOutWhenUnconnected=off
  wires:
  Mux/1 -> alfa/1, beta/1
  alfa/1 -> Mux1/1
  beta/1 -> Mux1/2
  Mux1/1 -> a/1, b/1, c/1
  a/1 -> Mux2/1
  b/1 -> Mux2/2
  c/1 -> Mux2/3
  dq/1 -> Mux/1
  sincos/1 -> Mux/2
  Mux2/1 -> abc/1

== system Grid_FormingVSG_PMSG/PMSM1/elemodel3/iq,id ==
  vd1,vq1 : Inport
  we : Inport  Port=2
  Flux : Inport  Port=3
  Demux : Demux  Outputs=2
  Mux : Mux  Inputs=2
  id : Subsystem
  iq : Subsystem
  id1,iq1 : Outport  InitialOutput=0  VectorParamsAs1DForOutWhenUnconnected=off
  wires:
  Mux/1 -> id1,iq1/1
  vd1,vq1/1 -> Demux/1
  Demux/1 -> id/1(vd1)
  Demux/2 -> iq/3(vq)
  id/1(id) -> iq/1(id), Mux/1
  we/1 -> iq/2(we), id/2(we)
  iq/1(iq) -> id/3(iq1), Mux/2
  Flux/1 -> iq/4(Flux)

== system Grid_FormingVSG_PMSG/PMSM1/elemodel3/sin(thr),cos(thr)1 ==
  thr : Inport
  Mux2 : Mux  Inputs=2
  Trigonometric Function : Trigonometry
  Trigonometric Function1 : Trigonometry  Operator=cos
  sin(thr),cos(thr) : Outport  OutputWhenDisabled=reset  InitialOutput=0  VectorParamsAs1DForOutWhenUnconnected=off
  wires:
  thr/1 -> Trigonometric Function1/1, Trigonometric Function/1  "thr"
  Mux2/1 -> sin(thr),cos(thr)/1
  Trigonometric Function1/1 -> Mux2/2
  Trigonometric Function/1 -> Mux2/1

== system Grid_FormingVSG_PMSG/PMSM1/elemodel3/abc to dq/Stationary reference frame ==
  ab : Inport
  Mux3 : Mux  Inputs=2
  d : Fcn  Expr=u(4)*u(1)+u(3)*u(2)
  q : Fcn  Expr=-u(3)*u(1)+u(4)*u(2)
  V_dq : Outport  OutputWhenDisabled=reset  InitialOutput=0  VectorParamsAs1DForOutWhenUnconnected=off
  wires:
  d/1 -> Mux3/1
  q/1 -> Mux3/2
  ab/1 -> d/1, q/1
  Mux3/1 -> V_dq/1
  ? -> ?

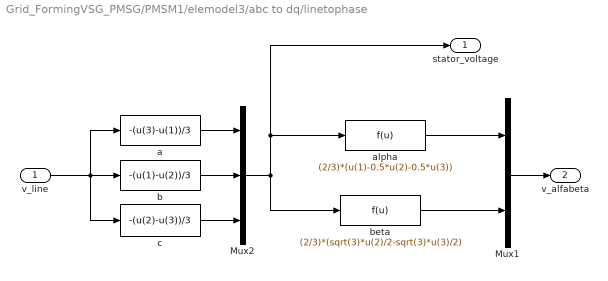
== system Grid_FormingVSG_PMSG/PMSM1/elemodel3/abc to dq/linetophase ==
  v_line : Inport
  Mux1 : Mux  Inputs=2
  Mux2 : Mux  Inputs=3
  a : Fcn  Expr=-(u(3)-u(1))/3
  alpha : Fcn  Expr=(2/3)*(u(1)-0.5*u(2)-0.5*u(3))
  b : Fcn  Expr=-(u(1)-u(2))/3
  beta : Fcn  Expr=(2/3)*(sqrt(3)*u(2)/2-sqrt(3)*u(3)/2)
  c : Fcn  Expr=-(u(2)-u(3))/3
  stator_voltage : Outport  VectorParamsAs1DForOutWhenUnconnected=off
  v_alfabeta : Outport  Port=2  VectorParamsAs1DForOutWhenUnconnected=off
  wires:
  a/1 -> Mux2/1
  b/1 -> Mux2/2
  c/1 -> Mux2/3
  v_line/1 -> b/1, a/1, c/1
  Mux2/1 -> beta/1, alpha/1, stator_voltage/1
  alpha/1 -> Mux1/1
  beta/1 -> Mux1/2
  Mux1/1 -> v_alfabeta/1

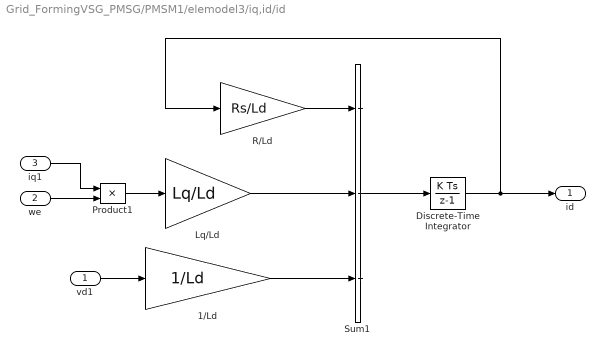
== system Grid_FormingVSG_PMSG/PMSM1/elemodel3/iq,id/id ==
  vd1 : Inport
  we : Inport  Port=2
  iq1 : Inport  Port=3
  1/Ld : Gain  Gain=1/Ld  SaturateOnIntegerOverflow=on  OutDataTypeStr=Inherit: Same as input  ParamDataTypeStr=Inherit: Same as input
  Discrete-Time Integrator : DiscreteIntegrator  SampleTime=Ts_step  ICPrevOutput=DiscIntNeverNeededParam  ICPrevScaledInput=DiscIntNeverNeededParam
  Lq/Ld : Gain  Gain=Lq/Ld  SaturateOnIntegerOverflow=on  OutDataTypeStr=Inherit: Same as input  ParamDataTypeStr=Inherit: Same as input
  Product1 : Product  InputSameDT=on  SaturateOnIntegerOverflow=on  OutDataTypeStr=Inherit: Same as first input
  R/Ld : Gain  Gain=Rs/Ld  SaturateOnIntegerOverflow=on  OutDataTypeStr=Inherit: Same as input  ParamDataTypeStr=Inherit: Same as input
  Sum1 : Sum  Inputs=-++  InputSameDT=on  SaturateOnIntegerOverflow=on  OutDataTypeStr=Inherit: Same as first input
  id : Outport  InitialOutput=0  VectorParamsAs1DForOutWhenUnconnected=off
  wires:
  R/Ld/1 -> Sum1/1
  Sum1/1 -> Discrete-Time Integrator/1
  Product1/1 -> Lq/Ld/1
  iq1/1 -> Product1/1
  vd1/1 -> 1/Ld/1
  we/1 -> Product1/2
  Discrete-Time Integrator/1 -> id/1, R/Ld/1
  Lq/Ld/1 -> Sum1/2
  1/Ld/1 -> Sum1/3

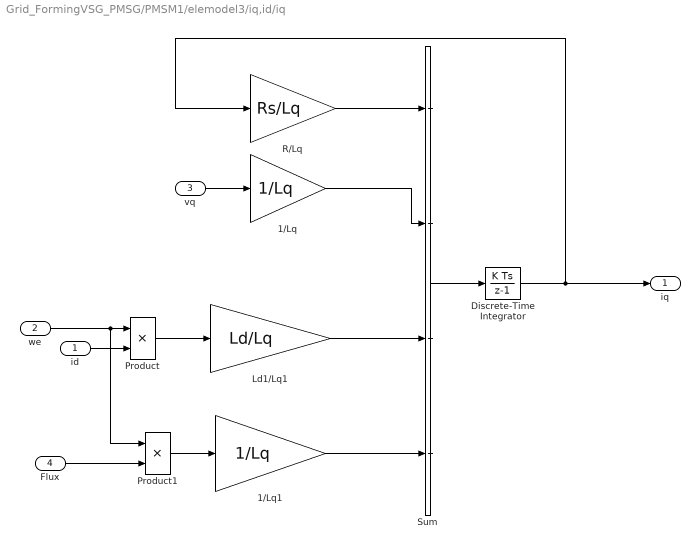
== system Grid_FormingVSG_PMSG/PMSM1/elemodel3/iq,id/iq ==
  id : Inport
  we : Inport  Port=2
  vq : Inport  Port=3
  Flux : Inport  Port=4
  1/Lq : Gain  Gain=1/Lq  SaturateOnIntegerOverflow=on  OutDataTypeStr=Inherit: Same as input  ParamDataTypeStr=Inherit: Same as input
  1/Lq1 : Gain  Gain=1/Lq  SaturateOnIntegerOverflow=on  OutDataTypeStr=Inherit: Same as input  ParamDataTypeStr=Inherit: Same as input
  Discrete-Time Integrator : DiscreteIntegrator  SampleTime=Ts_step  ICPrevOutput=DiscIntNeverNeededParam  ICPrevScaledInput=DiscIntNeverNeededParam
  Ld1/Lq1 : Gain  Gain=Ld/Lq  SaturateOnIntegerOverflow=on  OutDataTypeStr=Inherit: Same as input  ParamDataTypeStr=Inherit: Same as input
  Product : Product  InputSameDT=on  SaturateOnIntegerOverflow=on  OutDataTypeStr=Inherit: Same as first input
  Product1 : Product  InputSameDT=on  SaturateOnIntegerOverflow=on  OutDataTypeStr=Inherit: Same as first input
  R/Lq : Gain  Gain=Rs/Lq  SaturateOnIntegerOverflow=on  OutDataTypeStr=Inherit: Same as input  ParamDataTypeStr=Inherit: Same as input
  Sum : Sum  Inputs=-+--  InputSameDT=on  SaturateOnIntegerOverflow=on  OutDataTypeStr=Inherit: Same as first input
  iq : Outport  InitialOutput=0  VectorParamsAs1DForOutWhenUnconnected=off
  wires:
  R/Lq/1 -> Sum/1
  Sum/1 -> Discrete-Time Integrator/1
  Product/1 -> Ld1/Lq1/1
  Discrete-Time Integrator/1 -> iq/1, R/Lq/1
  vq/1 -> 1/Lq/1
  we/1 -> Product/1, Product1/1
  id/1 -> Product/2
  Product1/1 -> 1/Lq1/1
  Flux/1 -> Product1/2
  1/Lq/1 -> Sum/2
  Ld1/Lq1/1 -> Sum/3
  1/Lq1/1 -> Sum/4
